simulink model "longitudinal_stabilty"  (R2017b)
settings: Solver=VariableStepAuto  StartTime=0.0  StopTime=50  RelTol=1e-3
values from neighbouring files (symbols this model uses):
  A = A'    [c_l.m]    (also in c_m.m; c_n.m; c_x.m; c_z.m)
  B = ssm_b( state_trim, state_dot_trim, control_trim, xcg )    [ssm_f16.m]    (also in thrust.m = B')
  C = ssm_c( state_trim, state_dot_trim, control_trim, xcg )    [ssm_f16.m]    (also in thrust.m = C')
  control_trim = u0    [find_trim.m]
  D = ssm_d( state_trim, state_dot_trim, control_trim, xcg )    [ssm_f16.m]
libraries: F16_Actuator_Library x4
settings Model: Creator=monster  LastModifiedBy=monster

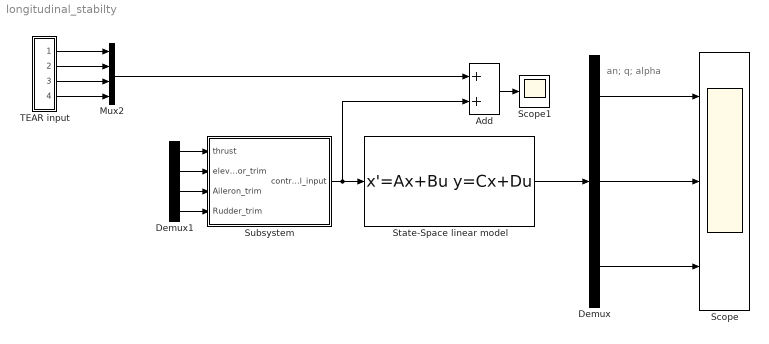
== system longitudinal_stabilty ==
  note: an;
      |
      | q;
      |
      | alpha
  Add : Sum
  Demux : Demux  Outputs=3
  Demux1 : Demux
  Mux2 : Mux
  Scope : Scope  NumInputPorts=3
  Scope1 : Scope
  "State-Space linear model " : StateSpace  A=A  B=B  C=C  D=D  InitialCondition=0
  Subsystem : Subsystem
  TEAR input : Subsystem
  wires:
  TEAR input/4(R) -> Mux2/4
  Demux1/1 -> Subsystem/1(thrust)
  TEAR input/2(E) -> Mux2/2
  TEAR input/1(T) -> Mux2/1
  Demux1/4 -> Subsystem/4(Rudder_trim)
  Demux1/3 -> Subsystem/3(Aileron_trim)
  Demux/3 -> Scope/3
  Add/1 -> Scope1/1
  "State-Space linear model "/1 -> Demux/1
  Demux/2 -> Scope/2
  Demux/1 -> Scope/1
  Subsystem/1(control_input) -> "State-Space linear model "/1, Add/2
  TEAR input/3(A) -> Mux2/3
  Mux2/1 -> Add/1
  Demux1/2 -> Subsystem/2(elevator_trim)

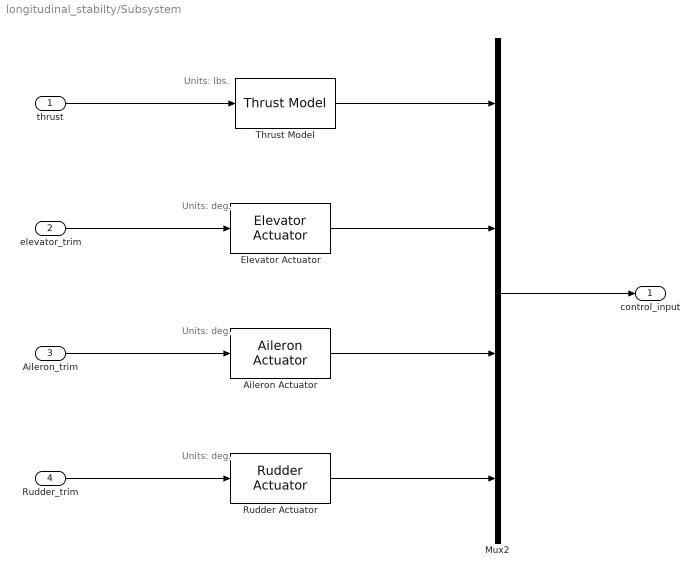
== system longitudinal_stabilty/Subsystem ==
  note: Units: deg.
  note: Units: deg.
  note: Units: lbs.
  note: Units: deg.
  thrust : Inport
  elevator_trim : Inport  Port=2
  Aileron_trim : Inport  Port=3
  Rudder_trim : Inport  Port=4
  Aileron Actuator : F16_Actuator_Library/Aileron Actuator
      link override "Integrator ": InitialCondition=0
  Elevator Actuator : F16_Actuator_Library/Elevator Actuator
      link override "Integrator ": InitialCondition=0
  Mux2 : Mux
  Rudder Actuator : F16_Actuator_Library/Rudder Actuator
      link override "Integrator ": InitialCondition=0
  Thrust Model : F16_Actuator_Library/Thrust Model
      link override "Integrator ": InitialCondition=0
  control_input : Outport
  wires:
  thrust/1 -> Thrust Model/1
  Aileron Actuator/1 -> Mux2/3
  Rudder_trim/1 -> Rudder Actuator/1
  Elevator Actuator/1 -> Mux2/2
  Rudder Actuator/1 -> Mux2/4
  elevator_trim/1 -> Elevator Actuator/1
  Aileron_trim/1 -> Aileron Actuator/1
  Thrust Model/1 -> Mux2/1
  Mux2/1 -> control_input/1

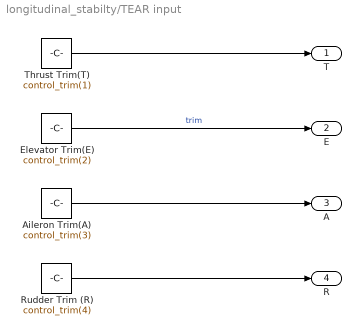
== system longitudinal_stabilty/TEAR input ==
  "Aileron Trim(A) " : Constant  Value=control_trim(3)
  "Elevator Trim(E) " : Constant  Value=control_trim(2)  VectorParams1D=off
  Rudder Trim (R) : Constant  Value=control_trim(4)
  "Thrust Trim(T) " : Constant  Value=control_trim(1)
  T : Outport
  E : Outport  Port=2
  A : Outport  Port=3
  R : Outport  Port=4
  wires:
  "Aileron Trim(A) "/1 -> A/1
  "Elevator Trim(E) "/1 -> E/1  "trim"
  "Thrust Trim(T) "/1 -> T/1
  Rudder Trim (R)/1 -> R/1
